simulink model "svlvvpr1_schema_system"  (R2020a)
settings: Solver=VariableStepAuto  StartTime=0.0  StopTime=10.0  RelTol=1e-3
settings Model: Creator=dot  LastModifiedBy=dot

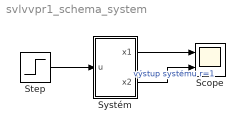
== system svlvvpr1_schema_system ==
  Scope : Scope  NumInputPorts=2
  Step : Step  SampleTime=0
  Systém : Subsystem
  wires:
  Step/1 -> Systém/1(u)
  Systém/1(x1) -> Scope/1
  Systém/2(x2) -> Scope/2  "výstup systému r=1"

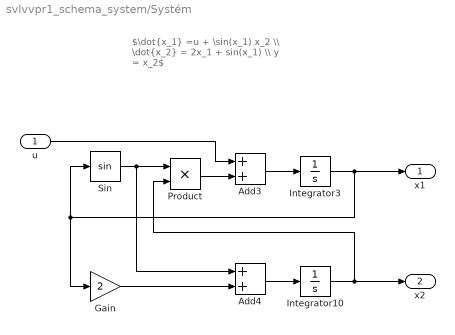
== system svlvvpr1_schema_system/Systém ==
  note: $\dot{x_1} =u + \sin(x_1) x_2 \\ \dot{x_2} = 2x_1 + sin(x_1) \\ y = x_2$
  u : Inport
  Add3 : Sum
  Add4 : Sum
  Gain : Gain  Gain=2
  Integrator10 : Integrator
  Integrator3 : Integrator
  Product : Product
  Sin : Trigonometry
  x1 : Outport
  x2 : Outport  Port=2
  wires:
  Add4/1 -> Integrator10/1
  Gain/1 -> Add4/2
  u/1 -> Add3/1
  Add3/1 -> Integrator3/1
  Integrator3/1 -> Sin/1, Gain/1, x1/1
  Product/1 -> Add3/2
  Integrator10/1 -> Product/2, x2/1
  Sin/1 -> Product/1, Add4/1
